simulink model "test"  (R2021a)
settings: Solver=VariableStepAuto  StartTime=0.0  StopTime=10.0  RelTol=1e-3
settings Model: Creator=ryusei  LastModifiedBy=ryusei
settings DataIOCC: InspectSignalLogs=on
settings SFSimCC: SimCustomSourceCode=|
  | >>clear
  | >>m=1; c=1; k=10;
  | >>whos

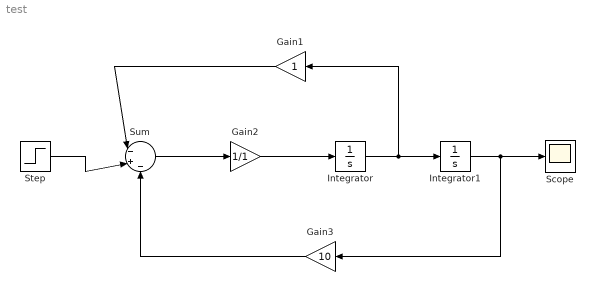
== system test ==
  Gain1 : Gain
  Gain2 : Gain  Gain=1/1
  Gain3 : Gain  Gain=10
  Integrator : Integrator
  Integrator1 : Integrator
  Scope : Scope
  Step : Step  SampleTime=0
  Sum : Sum  Inputs=|-+-
  wires:
  Step/1 -> Sum/2
  Gain1/1 -> Sum/1
  Sum/1 -> Gain2/1
  Gain2/1 -> Integrator/1
  Integrator/1 -> Gain1/1, Integrator1/1
  Integrator1/1 -> Gain3/1, Scope/1
  Gain3/1 -> Sum/3
